simulink model "Control_Model_2020a"  (R2020a)
settings: Solver=ode3  StartTime=0.0  StopTime=20  FixedStep=0.001  RelTol=1e-3
InitFcn:
  | init_parameters
undefined symbols (not defined in the file): Bf, Bm, Br, DiscIntNeverNeededParam, f, g, hg, i_sw, I_tire, Iz, k1, k2, k3, K_LQR, kd_beta, kd_omega, ki_beta, ki_omega, kp_beta, kp_omega, L, Lf, Lm, Lr, m, magnitude, mb, mw, Mz_K, Pn_motor, r, sigbuilder_block, Tn_motor, v_obj, vx0, w0
libraries: simulink x2, Solver_SF x1, simulink_extras x1
(part 2 of 2)

== system Control_Model_2020a/开环驾驶员模型/Sin_(后续可换为轨迹规划结果前向角) ==
  Clock : Clock
  Clock1 : Clock
  Constant : Constant  Value=0
  Constant1 : Constant  Value=0
  Scope : Scope
  Switch : Switch  Criteria=u2 > Threshold  Threshold=3
  Switch1 : Switch  Criteria=u2 > Threshold  Threshold=7
  Transport Delay1 : TransportDelay  DelayTime=3
  rad : Sin  Amplitude=2  Frequency=pi/2  SampleTime=0
  delta_sw : Outport
  wires:
  Constant1/1 -> Switch1/1
  Clock/1 -> Switch/2
  rad/1 -> Transport Delay1/1
  Switch1/1 -> delta_sw/1
  Clock1/1 -> Switch1/2
  Switch/1 -> Switch1/3
  Transport Delay1/1 -> Switch/1, Scope/1
  Constant/1 -> Switch/3

== system Control_Model_2020a/开环驾驶员模型/Step ==
  Step : Step  After=1.4  SampleTime=0
  delta_sw : Outport
  wires:
  Step/1 -> delta_sw/1

== system Control_Model_2020a/7DOF_vehicle/Body/global system transform ==
  vx : Inport
  vy : Inport  Port=2
  wz : Inport  Port=3
  Add : Sum  Inputs=|+-
  Add1 : Sum  Inputs=|++
  Integrator10 : Integrator
  Integrator8 : Integrator
  Integrator9 : Integrator
  Scope : Scope  NumInputPorts=3
  Trigonometric Function1 : Trigonometry
  Trigonometric Function2 : Trigonometry  Operator=cos
  vx*cosr : Product
  vx*sinr : Product
  vy*cosr : Product
  vy*sinr : Product
  x : Outport
  y : Outport  Port=2
  wires:
  vy*cosr/1 -> Add1/2
  Add1/1 -> Scope/2, Integrator9/1
  vx*sinr/1 -> Add1/1
  vx*cosr/1 -> Add/1
  Integrator8/1 -> Scope/1, Trigonometric Function1/1, Trigonometric Function2/1  "r"
  Integrator10/1 -> x/1
  Integrator9/1 -> y/1
  vy/1 -> vy*cosr/1, vy*sinr/1
  wz/1 -> Scope/3, Integrator8/1
  vx/1 -> vx*cosr/1, vx*sinr/1
  vy*sinr/1 -> Add/2
  Trigonometric Function2/1 -> vx*cosr/2, vy*cosr/2
  Add/1 -> Integrator10/1
  Trigonometric Function1/1 -> vx*sinr/2, vy*sinr/2

== system Control_Model_2020a/7DOF_vehicle/Wheel/fl ==
  T_fl : Inport
  Fx_fl : Inport  Port=2
  Fz_fl : Inport  Port=3
  Add : Sum  Inputs=+--
  Constant : Constant  Value=I_tire
  Divide : Product  Inputs=*/
  Gain : Gain  Gain=r
  Gain1 : Gain  Gain=r*f
  Integrator : Integrator  InitialCondition=w0
  w_fl : Outport
  wires:
  Gain/1 -> Add/2
  Fx_fl/1 -> Gain/1
  Fz_fl/1 -> Gain1/1
  T_fl/1 -> Add/1
  Gain1/1 -> Add/3
  Add/1 -> Divide/1
  Constant/1 -> Divide/2
  Divide/1 -> Integrator/1  "dot_w"
  Integrator/1 -> w_fl/1

== system Control_Model_2020a/7DOF_vehicle/Wheel/fr ==
  T_fr : Inport
  Fx_fr : Inport  Port=2
  Fz_fr : Inport  Port=3
  Add : Sum  Inputs=+--
  Constant : Constant  Value=I_tire
  Divide : Product  Inputs=*/
  Gain : Gain  Gain=r
  Gain1 : Gain  Gain=r*f
  Integrator : Integrator  InitialCondition=w0
  w_fr : Outport
  wires:
  Gain1/1 -> Add/3
  Integrator/1 -> w_fr/1
  Divide/1 -> Integrator/1  "dot_w"
  Constant/1 -> Divide/2
  Add/1 -> Divide/1
  Gain/1 -> Add/2
  T_fr/1 -> Add/1
  Fz_fr/1 -> Gain1/1
  Fx_fr/1 -> Gain/1

== system Control_Model_2020a/7DOF_vehicle/Wheel/ml ==
  T_ml : Inport
  Fx_ml : Inport  Port=2
  Fz_ml : Inport  Port=3
  Add : Sum  Inputs=+--
  Constant : Constant  Value=I_tire
  Divide : Product  Inputs=*/
  Gain : Gain  Gain=r
  Gain1 : Gain  Gain=r*f
  Integrator : Integrator  InitialCondition=w0
  w_ml : Outport
  wires:
  Fx_ml/1 -> Gain/1
  Fz_ml/1 -> Gain1/1
  T_ml/1 -> Add/1
  Gain/1 -> Add/2
  Add/1 -> Divide/1
  Constant/1 -> Divide/2
  Divide/1 -> Integrator/1  "dot_w"
  Integrator/1 -> w_ml/1
  Gain1/1 -> Add/3

== system Control_Model_2020a/7DOF_vehicle/Wheel/mr ==
  T_mr : Inport
  Fx_mr : Inport  Port=2
  Fz_mr : Inport  Port=3
  Add : Sum  Inputs=+--
  Constant : Constant  Value=I_tire
  Divide : Product  Inputs=*/
  Gain : Gain  Gain=r
  Gain1 : Gain  Gain=r*f
  Integrator : Integrator  InitialCondition=w0
  w_mr : Outport
  wires:
  Integrator/1 -> w_mr/1
  Divide/1 -> Integrator/1  "dot_w"
  Constant/1 -> Divide/2
  Add/1 -> Divide/1
  Gain/1 -> Add/2
  T_mr/1 -> Add/1
  Fz_mr/1 -> Gain1/1
  Fx_mr/1 -> Gain/1
  Gain1/1 -> Add/3

== system Control_Model_2020a/7DOF_vehicle/Wheel/rl ==
  T_rl : Inport
  Fx_rl : Inport  Port=2
  Fz_rl : Inport  Port=3
  Add : Sum  Inputs=+--
  Constant : Constant  Value=I_tire
  Divide : Product  Inputs=*/
  Gain : Gain  Gain=r
  Gain1 : Gain  Gain=r*f
  Integrator : Integrator  InitialCondition=w0
  w_rl : Outport
  wires:
  Gain1/1 -> Add/3
  Integrator/1 -> w_rl/1
  Divide/1 -> Integrator/1  "dot_w"
  Constant/1 -> Divide/2
  Add/1 -> Divide/1
  Gain/1 -> Add/2
  T_rl/1 -> Add/1
  Fz_rl/1 -> Gain1/1
  Fx_rl/1 -> Gain/1

== system Control_Model_2020a/7DOF_vehicle/Wheel/rr ==
  T_rr : Inport
  Fx_rr : Inport  Port=2
  Fz_rr : Inport  Port=3
  Add : Sum  Inputs=+--
  Constant : Constant  Value=I_tire
  Divide : Product  Inputs=*/
  Gain : Gain  Gain=r
  Gain1 : Gain  Gain=r*f
  Integrator : Integrator  InitialCondition=w0
  w_rr : Outport
  wires:
  Gain1/1 -> Add/3
  Fx_rr/1 -> Gain/1
  Fz_rr/1 -> Gain1/1
  T_rr/1 -> Add/1
  Gain/1 -> Add/2
  Add/1 -> Divide/1
  Constant/1 -> Divide/2
  Divide/1 -> Integrator/1  "dot_w"
  Integrator/1 -> w_rr/1

== system Control_Model_2020a/7DOF_vehicle/alpha_lamda/alpha ==
  vx : Inport
  vy : Inport  Port=2
  wz : Inport  Port=3
  delta_fl : Inport  Port=4
  delta_fr : Inport  Port=5
  Gain{,1..5} (6 alike) : Gain  Gain=-1
  fl : Subsystem
  fr : Subsystem
  ml : Subsystem
  mr : Subsystem
  rl : Subsystem
  rr : Subsystem
  alpha_fl : Outport
  alpha_fr : Outport  Port=2
  alpha_rl : Outport  Port=3
  alpha_rr : Outport  Port=4
  alpha_ml : Outport  Port=5
  alpha_mr : Outport  Port=6
  wires:
  delta_fr/1 -> fr/4(delta_fr)
  delta_fl/1 -> fl/4(delta_fl)
  vy/1 -> rl/2(vy), mr/2(vy), ml/2(vy), fl/2(vy), fr/2(vy), rr/2(vy)
  vx/1 -> rl/1(vx), mr/1(vx), ml/1(vx), fl/1(vx), fr/1(vx), rr/1(vx)
  wz/1 -> rl/3(wz), fr/3(wz), rr/3(wz), mr/3(wz), ml/3(wz), fl/3(wz)
  fl/1(alpha_fl) -> Gain/1
  Gain/1 -> alpha_fl/1
  rl/1(alpha_rl) -> Gain1/1
  Gain1/1 -> alpha_rl/1
  fr/1(alpha_fr) -> Gain2/1
  Gain2/1 -> alpha_fr/1
  rr/1(alpha_rr) -> Gain3/1
  Gain3/1 -> alpha_rr/1
  Gain4/1 -> alpha_ml/1
  Gain5/1 -> alpha_mr/1
  ml/1(alpha_ml) -> Gain4/1
  mr/1(alpha_mr) -> Gain5/1

== system Control_Model_2020a/7DOF_vehicle/alpha_lamda/lamda ==
  vx : Inport
  vy : Inport  Port=2
  wz : Inport  Port=3
  delta_fl : Inport  Port=4
  delta_fr : Inport  Port=5
  w_fl : Inport  Port=6
  w_fr : Inport  Port=7
  w_rl : Inport  Port=8
  w_rr : Inport  Port=9
  w_ml : Inport  Port=10
  w_mr : Inport  Port=11
  fl : Subsystem
  fr : Subsystem
  ml : Subsystem
  mr : Subsystem
  rl : Subsystem
  rr : Subsystem
  lamda_fl : Outport
  lamda_fr : Outport  Port=2
  lamda_rl : Outport  Port=3
  lamda_rr : Outport  Port=4
  lamda_ml : Outport  Port=5
  lamda_mr : Outport  Port=6
  wires:
  fr/1(lamda_fr) -> lamda_fr/1
  rr/1(lamda_rr) -> lamda_rr/1
  w_rl/1 -> rl/1(w_rl)
  w_rr/1 -> rr/1(w_rr)
  w_fr/1 -> fr/1(w_fr)
  delta_fr/1 -> fr/5(delta_fr)
  delta_fl/1 -> fl/5(delta_fl)
  vy/1 -> fl/4(vy), fr/4(vy)
  vx/1 -> fl/3(vx), fr/3(vx), mr/3(vx), rr/3(vx), ml/3(vx), rl/3(vx)
  wz/1 -> fl/2(wz), fr/2(wz), mr/2(wz), rr/2(wz), ml/2(wz), rl/2(wz)
  w_fl/1 -> fl/1(w_fl)
  rl/1(lamda_rl) -> lamda_rl/1
  fl/1(lamda_fl) -> lamda_fl/1
  w_ml/1 -> ml/1(w_ml)
  w_mr/1 -> mr/1(w_mr)
  ml/1(lamda_ml) -> lamda_ml/1
  mr/1(lamda_mr) -> lamda_mr/1

== system Control_Model_2020a/开环驾驶员模型/Sin/Signal Builder ==
  Demux : Demux  Tag=STV Demux  Outputs=1
      settings: DisplayOption=none
  FromWs : FromWorkspace  Tag=STV FromWs  VariableName=tuvar
      SigBuilderData=|
      | common.afterFinalStr = 'Extrapolate'
      | common.sampleTime = 0
      | dataSet.timeRange = [0 10]
      | dataSet.name = 'Group 1'
      | sbobj.Groups.Name = 'Group 1'
      | sbobj.Groups.Signals.Name = 'Signal 1'
      | sbobj.Groups.Signals.XData = [0 1 1.55 2 3 10]
      | sbobj.Groups.Signals.YData = [0 0 294 294 -294 -294]
  Signal 1 : Outport  Tag=STV Outport
  wires:
  Demux/1 -> Signal 1/1
  FromWs/1 -> Demux/1

== system Control_Model_2020a/7DOF_vehicle/alpha_lamda/alpha/fl ==
  vx : Inport
  vy : Inport  Port=2
  wz : Inport  Port=3
  delta_fl : Inport  Port=4
  Add2 : Sum
  Add3 : Sum  Inputs=+-
  Add4 : Sum  Inputs=-+
  Divide : Product  Inputs=/*
  Gain3 : Gain  Gain=Lf
  Gain4 : Gain  Gain=0.5*Bf
  Trigonometric Function : Trigonometry  Operator=atan
  alpha_fl : Outport
  wires:
  wz/1 -> Gain3/1, Gain4/1
  Add4/1 -> alpha_fl/1
  vy/1 -> Add2/1
  delta_fl/1 -> Add4/2
  vx/1 -> Add3/1
  Trigonometric Function/1 -> Add4/1
  Divide/1 -> Trigonometric Function/1
  Add3/1 -> Divide/1
  Add2/1 -> Divide/2
  Gain4/1 -> Add3/2
  Gain3/1 -> Add2/2

== system Control_Model_2020a/7DOF_vehicle/alpha_lamda/alpha/fr ==
  vx : Inport
  vy : Inport  Port=2
  wz : Inport  Port=3
  delta_fr : Inport  Port=4
  Add2 : Sum
  Add3 : Sum
  Add4 : Sum  Inputs=-+
  Divide : Product  Inputs=/*
  Gain3 : Gain  Gain=Lf
  Gain4 : Gain  Gain=0.5*Bf
  Trigonometric Function : Trigonometry  Operator=atan
  alpha_fr : Outport
  wires:
  Gain3/1 -> Add2/2
  Add2/1 -> Divide/2
  Add3/1 -> Divide/1
  Divide/1 -> Trigonometric Function/1
  Trigonometric Function/1 -> Add4/1
  vx/1 -> Add3/1
  delta_fr/1 -> Add4/2
  vy/1 -> Add2/1
  Add4/1 -> alpha_fr/1
  wz/1 -> Gain4/1, Gain3/1
  Gain4/1 -> Add3/2

== system Control_Model_2020a/7DOF_vehicle/alpha_lamda/alpha/ml ==
  vx : Inport
  vy : Inport  Port=2
  wz : Inport  Port=3
  Add2 : Sum  Inputs=+-
  Add3 : Sum  Inputs=+-
  Divide : Product  Inputs=/*
  Gain1 : Gain  Gain=-1
  Gain3 : Gain  Gain=Lm
  Gain4 : Gain  Gain=0.5*Bm
  Trigonometric Function : Trigonometry  Operator=atan
  alpha_ml : Outport
  wires:
  Gain1/1 -> alpha_ml/1
  Gain4/1 -> Add3/2
  Trigonometric Function/1 -> Gain1/1
  wz/1 -> Gain3/1, Gain4/1
  vy/1 -> Add2/1
  vx/1 -> Add3/1
  Divide/1 -> Trigonometric Function/1
  Add3/1 -> Divide/1
  Add2/1 -> Divide/2
  Gain3/1 -> Add2/2

== system Control_Model_2020a/7DOF_vehicle/alpha_lamda/alpha/mr ==
  vx : Inport
  vy : Inport  Port=2
  wz : Inport  Port=3
  Add2 : Sum  Inputs=+-
  Add3 : Sum
  Divide : Product  Inputs=/*
  Gain2 : Gain  Gain=-1
  Gain3 : Gain  Gain=Lm
  Gain4 : Gain  Gain=0.5*Bm
  Trigonometric Function : Trigonometry  Operator=atan
  alpha_mr : Outport
  wires:
  Gain2/1 -> alpha_mr/1
  Gain4/1 -> Add3/2
  Gain3/1 -> Add2/2
  Add2/1 -> Divide/2
  Add3/1 -> Divide/1
  Divide/1 -> Trigonometric Function/1
  vx/1 -> Add3/1
  vy/1 -> Add2/1
  wz/1 -> Gain4/1, Gain3/1
  Trigonometric Function/1 -> Gain2/1

== system Control_Model_2020a/7DOF_vehicle/alpha_lamda/alpha/rl ==
  vx : Inport
  vy : Inport  Port=2
  wz : Inport  Port=3
  Add2 : Sum  Inputs=+-
  Add3 : Sum  Inputs=+-
  Divide : Product  Inputs=/*
  Gain1 : Gain  Gain=-1
  Gain3 : Gain  Gain=Lr
  Gain4 : Gain  Gain=0.5*Br
  Trigonometric Function : Trigonometry  Operator=atan
  alpha_rl : Outport
  wires:
  Gain3/1 -> Add2/2
  Add2/1 -> Divide/2
  Add3/1 -> Divide/1
  Divide/1 -> Trigonometric Function/1
  vx/1 -> Add3/1
  vy/1 -> Add2/1
  wz/1 -> Gain4/1, Gain3/1
  Trigonometric Function/1 -> Gain1/1
  Gain4/1 -> Add3/2
  Gain1/1 -> alpha_rl/1

== system Control_Model_2020a/7DOF_vehicle/alpha_lamda/alpha/rr ==
  vx : Inport
  vy : Inport  Port=2
  wz : Inport  Port=3
  Add2 : Sum  Inputs=+-
  Add3 : Sum
  Divide : Product  Inputs=/*
  Gain2 : Gain  Gain=-1
  Gain3 : Gain  Gain=Lr
  Gain4 : Gain  Gain=0.5*Br
  Trigonometric Function : Trigonometry  Operator=atan
  alpha_rr : Outport
  wires:
  Trigonometric Function/1 -> Gain2/1
  wz/1 -> Gain3/1, Gain4/1
  vy/1 -> Add2/1
  vx/1 -> Add3/1
  Divide/1 -> Trigonometric Function/1
  Add3/1 -> Divide/1
  Add2/1 -> Divide/2
  Gain3/1 -> Add2/2
  Gain4/1 -> Add3/2
  Gain2/1 -> alpha_rr/1

== system Control_Model_2020a/7DOF_vehicle/alpha_lamda/lamda/fl ==
  w_fl : Inport
  wz : Inport  Port=2
  vx : Inport  Port=3
  vy : Inport  Port=4
  delta_fl : Inport  Port=5
  Add1 : Sum  Inputs=-+
  Add2 : Sum
  Add3 : Sum
  Add4 : Sum  Inputs=+-
  Constant1 : Constant  Value=r
  Divide1 : Product  Inputs=**
  Divide2 : Product  Inputs=**
  Divide3 : Product  Inputs=**
  Divide4 : Product  Inputs=/*
  Divide5 : Product  Inputs=*/
  Fcn1 : Fcn  Expr=u+(u==0)*eps
  Gain2 : Gain  Gain=0.5*Bf
  Gain3 : Gain  Gain=Lf
  Saturation : Saturate  UpperLimit=1  LowerLimit=-1
  Switch : Switch  Criteria=u2 > Threshold
  Trigonometric Function1 : Trigonometry
  Trigonometric Function2 : Trigonometry  Operator=cos
  lamda_fl : Outport
  wires:
  Switch/1 -> Saturation/1
  Add3/1 -> Add4/2, Divide5/2  "Vwx_fl"
  Add4/1 -> Switch/2, Divide4/2, Divide5/1
  Divide4/1 -> Switch/1
  Divide5/1 -> Switch/3
  Fcn1/1 -> Divide4/1
  vx/1 -> Add1/2
  Gain2/1 -> Add1/1
  wz/1 -> Gain3/1, Gain2/1
  Add1/1 -> Divide1/1
  delta_fl/1 -> Trigonometric Function2/1, Trigonometric Function1/1
  Trigonometric Function2/1 -> Divide1/2
  vy/1 -> Add2/2
  Gain3/1 -> Add2/1
  Add2/1 -> Divide2/1
  Trigonometric Function1/1 -> Divide2/2
  Divide1/1 -> Add3/1
  Divide2/1 -> Add3/2
  w_fl/1 -> Divide3/1
  Constant1/1 -> Divide3/2
  Divide3/1 -> Add4/1, Fcn1/1  "w*I_tire"
  Saturation/1 -> lamda_fl/1

== system Control_Model_2020a/7DOF_vehicle/alpha_lamda/lamda/fr ==
  w_fr : Inport
  wz : Inport  Port=2
  vx : Inport  Port=3
  vy : Inport  Port=4
  delta_fr : Inport  Port=5
  Add1 : Sum
  Add2 : Sum
  Add3 : Sum
  Add4 : Sum  Inputs=+-
  Constant1 : Constant  Value=r
  Divide1 : Product  Inputs=**
  Divide2 : Product  Inputs=**
  Divide3 : Product  Inputs=**
  Divide4 : Product  Inputs=/*
  Divide5 : Product  Inputs=*/
  Fcn1 : Fcn  Expr=u+(u==0)*eps
  Gain2 : Gain  Gain=0.5*Bf
  Gain3 : Gain  Gain=Lf
  Saturation : Saturate  UpperLimit=1  LowerLimit=-1
  Switch : Switch  Criteria=u2 > Threshold
  Trigonometric Function1 : Trigonometry
  Trigonometric Function2 : Trigonometry  Operator=cos
  lamda_fr : Outport
  wires:
  Saturation/1 -> lamda_fr/1
  vx/1 -> Add1/2
  Gain2/1 -> Add1/1
  wz/1 -> Gain3/1, Gain2/1
  Add1/1 -> Divide1/1
  delta_fr/1 -> Trigonometric Function2/1, Trigonometric Function1/1
  Trigonometric Function2/1 -> Divide1/2
  vy/1 -> Add2/2
  Gain3/1 -> Add2/1
  Add2/1 -> Divide2/1
  Trigonometric Function1/1 -> Divide2/2
  Divide1/1 -> Add3/1
  Divide2/1 -> Add3/2
  w_fr/1 -> Divide3/1
  Constant1/1 -> Divide3/2
  Divide3/1 -> Fcn1/1, Add4/1  "w*I_tire"
  Fcn1/1 -> Divide4/1
  Divide5/1 -> Switch/3
  Divide4/1 -> Switch/1
  Add4/1 -> Divide5/1, Divide4/2, Switch/2
  Add3/1 -> Divide5/2, Add4/2  "Vwx_fr"
  Switch/1 -> Saturation/1

== system Control_Model_2020a/7DOF_vehicle/alpha_lamda/lamda/ml ==
  w_ml : Inport
  wz : Inport  Port=2
  vx : Inport  Port=3
  Add1 : Sum  Inputs=-+
  Add4 : Sum  Inputs=+-
  Constant1 : Constant  Value=r
  Divide3 : Product  Inputs=**
  Divide4 : Product  Inputs=/*
  Divide5 : Product  Inputs=*/
  Fcn1 : Fcn  Expr=u+(u==0)*eps
  Gain2 : Gain  Gain=0.5*Bm
  Saturation : Saturate  UpperLimit=1  LowerLimit=-1
  Switch : Switch  Criteria=u2 > Threshold
  lamda_ml : Outport
  wires:
  Switch/1 -> Saturation/1
  Add1/1 -> Add4/2, Divide5/2
  Add4/1 -> Switch/2, Divide4/2, Divide5/1
  Divide4/1 -> Switch/1
  Divide5/1 -> Switch/3
  Fcn1/1 -> Divide4/1
  Divide3/1 -> Add4/1, Fcn1/1  "w*I_tire"
  Constant1/1 -> Divide3/2
  w_ml/1 -> Divide3/1
  wz/1 -> Gain2/1
  Gain2/1 -> Add1/1
  vx/1 -> Add1/2
  Saturation/1 -> lamda_ml/1

== system Control_Model_2020a/7DOF_vehicle/alpha_lamda/lamda/mr ==
  w_mr : Inport
  wz : Inport  Port=2
  vx : Inport  Port=3
  Add1 : Sum
  Add4 : Sum  Inputs=+-
  Constant1 : Constant  Value=r
  Divide3 : Product  Inputs=**
  Divide4 : Product  Inputs=/*
  Divide5 : Product  Inputs=*/
  Fcn1 : Fcn  Expr=u+(u==0)*eps
  Gain2 : Gain  Gain=0.5*Bm
  Saturation : Saturate  UpperLimit=1  LowerLimit=-1
  Switch : Switch  Criteria=u2 > Threshold
  lamda_mr : Outport
  wires:
  Add1/1 -> Add4/2, Divide5/2  "Vwx_mr"
  Add4/1 -> Switch/2, Divide4/2, Divide5/1
  Divide4/1 -> Switch/1
  Divide5/1 -> Switch/3
  Fcn1/1 -> Divide4/1
  Divide3/1 -> Add4/1, Fcn1/1  "w*I_tire"
  vx/1 -> Add1/2
  Gain2/1 -> Add1/1
  wz/1 -> Gain2/1
  w_mr/1 -> Divide3/1
  Constant1/1 -> Divide3/2
  Switch/1 -> Saturation/1
  Saturation/1 -> lamda_mr/1

== system Control_Model_2020a/7DOF_vehicle/alpha_lamda/lamda/rl ==
  w_rl : Inport
  wz : Inport  Port=2
  vx : Inport  Port=3
  Add1 : Sum  Inputs=-+
  Add4 : Sum  Inputs=+-
  Constant1 : Constant  Value=r
  Divide3 : Product  Inputs=**
  Divide4 : Product  Inputs=/*
  Divide5 : Product  Inputs=*/
  Fcn1 : Fcn  Expr=u+(u==0)*eps
  Gain2 : Gain  Gain=0.5*Br
  Saturation : Saturate  UpperLimit=1  LowerLimit=-1
  Switch : Switch  Criteria=u2 > Threshold
  lamda_rl : Outport
  wires:
  Saturation/1 -> lamda_rl/1
  vx/1 -> Add1/2
  Gain2/1 -> Add1/1
  wz/1 -> Gain2/1
  w_rl/1 -> Divide3/1
  Constant1/1 -> Divide3/2
  Divide3/1 -> Fcn1/1, Add4/1  "w*I_tire"
  Fcn1/1 -> Divide4/1
  Divide5/1 -> Switch/3
  Divide4/1 -> Switch/1
  Add4/1 -> Divide5/1, Divide4/2, Switch/2
  Add1/1 -> Divide5/2, Add4/2
  Switch/1 -> Saturation/1

== system Control_Model_2020a/7DOF_vehicle/alpha_lamda/lamda/rr ==
  w_rr : Inport
  wz : Inport  Port=2
  vx : Inport  Port=3
  Add1 : Sum
  Add4 : Sum  Inputs=+-
  Constant1 : Constant  Value=r
  Divide3 : Product  Inputs=**
  Divide4 : Product  Inputs=/*
  Divide5 : Product  Inputs=*/
  Fcn1 : Fcn  Expr=u+(u==0)*eps
  Gain2 : Gain  Gain=0.5*Br
  Saturation : Saturate  UpperLimit=1  LowerLimit=-1
  Switch : Switch  Criteria=u2 > Threshold
  lamda_rr : Outport
  wires:
  Saturation/1 -> lamda_rr/1
  Switch/1 -> Saturation/1
  Constant1/1 -> Divide3/2
  w_rr/1 -> Divide3/1
  wz/1 -> Gain2/1
  Gain2/1 -> Add1/1
  vx/1 -> Add1/2
  Divide3/1 -> Fcn1/1, Add4/1  "w*I_tire"
  Fcn1/1 -> Divide4/1
  Divide5/1 -> Switch/3
  Divide4/1 -> Switch/1
  Add4/1 -> Divide5/1, Divide4/2, Switch/2
  Add1/1 -> Divide5/2, Add4/2  "Vwx_rr"

== matlab function Control_Model_2020a/Subsystem/Union_Control/MATLAB Function1 ==
  data: u input; B1 output; B2 output
function [B1,B2] = Param_B1B2(u)
if u>=0 && u<0.2
    B1=0.284;B2=2.577;
elseif u>=0.2 && u<0.4
    B1=0.297;B2=3.345;
elseif u>=0.4 && u<0.6
    B1=0.303;B2=4.228;
elseif u>=0.6 && u<0.8
    B1=0.357;B2=4.654;
else 
    B1=0.357;B2=5.573;
end

== matlab function Control_Model_2020a/average_control1/MATLAB Function1 ==
  data: Fz_fl input; Fz_fr input; Fz_rl input; T_fl output; Fz_rr input; T_vx input; M_yaw input; r input; Br input; T_fr output; T_rl output; T_rr output
function [T_fl,T_fr,T_rl,T_rr] = Optimal(Fz_fl,Fz_fr,Fz_rl,Fz_rr,T_vx,M_yaw,r,Br)

T_fl=T_vx/4-M_yaw*r/2/3.2;
T_fr=T_vx/4+M_yaw*r/2/3.2;
T_rl=T_vx/4-M_yaw*r/2/3.2;
T_rr=T_vx/4+M_yaw*r/2/3.2;

== matlab function Control_Model_2020a/Subsystem/Controller_wz/MATLAB Function1 ==
  data: x input; M output
function M=sat(x)
k=5;
d=abs(x/k);
if d<=1
M=x/k;
else
M=sign(x/k);
end

== matlab function Control_Model_2020a/Subsystem/Controller_beta/MATLAB Function1 ==
  data: x input; M output
function M=sat(x)
k=2;
d=abs(x/k);
if d<=1
M=x/k;
else
M=sign(x/k);
end

== matlab function Control_Model_2020a/MPC_Controller/MATLAB Function ==
  data: x input size=[8,1]; delta_u output
function delta_u = fcn(x)
Np =20;     % 预测时域
Nc = 20;     % 控制时域
x_num = 2; % 状态量的个数
u_num = 1; % 控制量的个数
% 参数值，包括：
% 前轴距离质心长度 lf   m
% 后轴距离质心长度 lr   m
% 整车质量 m    kg
% 横摆转动惯量 Iz kg*m^2
lf = 1.02;lr=1.89;m = 1412;Iz=1536.7;
% 前后轴轮胎侧偏刚度 Cf 和 Cr
Cf = -43214*2;Cr = -43214*2;
% 质心侧偏角 x(1)    rad
beta = x(1);
% 横摆角速度 x(2)    rad/s
omega = x(2);
% 前轮转角   x(3)    rad       
delta = x(3);
% 纵向车速 u         m/s
u = x(4);
% 上一周期控制量
u_k_1 = x(8);
% MPC 控制中的状态量与控制量集合
ksi = [beta;omega;u_k_1];

% 二自由度动力学方程得到系统状态转移矩阵 A
a11 = (Cf+Cr)./m/u;
a12 = (Cf*lf-Cr*lr)./m/u^2 - 1;
a21 = (Cf*lf-Cr*lr)./Iz;
a22 = (lf^2*Cf+lr^2*Cr)./Iz/u;

b11 = -Cf/m/u; % *(cos(delta)-delta*sin(delta))
b21 = -lf*Cf/Iz;
A = [a11 a12;a21 a22];
B = [0;1/Iz];
Bcd = [b11;b21];
% 采样时间
T = x(7);
rank = length(A);
% 时间步长 T 进行离散化
G = T*A + eye(rank);
H = T*B;
Bd = T*Bcd;
% 将状态与控制量集合后的增广矩阵
A_ = [G H;zeros(1,2) eye(1)];
B_ = [H;eye(1)];
C_ = [eye(2) zeros(2,1)];
Bd_ = [Bd;0];
% 开始构造 MPC 矩阵（具体原理查看说明文档）
% 构造 MPC 中的 Sc 矩阵（具体原理查看说明文档）
Sc = zeros(Np*x_num,x_num+1);
for i = 1:Np
    Sc((x_num*(i-1)+1):x_num*i,:) = C_*(A_^i);
end
% 构造 MPC 中的 Sd 矩阵（具体原理查看说明文档）
tmp = zeros(x_num,1);
Sd = zeros(Np*x_num,1);
for i = 1:Np
    tmp = tmp + C_*(A_^(i-1))*Bd_;
    Sd((x_num*(i-1)+1):x_num*i) = tmp;
end
% 构造 MPC 中的 Su 矩阵（具体原理查看说明文档）
Su = zeros(Np*x_num,Nc);
for i = 1:Np
    Su_tmp = zeros(x_num,Nc);
    zero_tmp = zeros(x_num,1);
    for j = 1:Nc
        if j<=i
            Su_tmp(:,j) = C_*(A_^(i-j))*B_;
        else
            Su_tmp(:,j) = zero_tmp;
        end
    end
    Su((x_num*(i-1)+1):x_num*i,:) = Su_tmp;
end

% Q 矩阵（权重系数）（具体原理查看说明文档）
Q = zeros(Np*x_num,Np*x_num);
Qi = [0 0;0 10];
zero_tmp = zeros(x_num,x_num);
for i = 1:Np
    Q_tmp = zeros(x_num,Np*x_num);
    for j = 1:Np
        if j==i
            Q_tmp(:,(x_num*(j-1)+1):x_num*j) = Qi;
        else
            Q_tmp(:,(x_num*(j-1)+1):x_num*j) = zero_tmp;
        end
    end
    Q((x_num*(i-1)+1):x_num*i,:) = Q_tmp;
end
% 质心侧偏角与横摆角速度参考值 x(5) 与 x(6)
beta_ref = x(5);
omega_ref = x(6);
Ri = [beta_ref;omega_ref];
Ref = zeros(Np*x_num,1);
% 将当前时刻的参考值设置为整个预测时域内的参考值（可修改为递增模式等）
for i = 1:Np
    %     Ref((2*(i-1)+1):2*i,:) = R_current + (Ri - R_current) * (i/Np);
    Ref((2*(i-1)+1):2*i,:) = Ri; % 期望为恒定值
end
% 计算 MPC 中的关键矩阵
E = Sc*ksi+Sd*delta-Ref;
R = 0.0003*eye(Nc);
H = 2*(Su'*Q'*Q*Su + R'*R);
G = 2*E'*Q'*Q*Su;
% J = 1/2*delta_u'*H*delta_u + G*delta_u;
% 这里用的无约束快速求解方法
% delta_u_arr = zeros(Nm,1);
% [delta_u_arr,~]=quadprog(H,G,[],[]);%计算得到delta_u(m)
%%
delta_u_arr = zeros(Nc,1);
% -inv(H)*G' 直接调用 MPC 简化求解方法，得到控制量
delta_u_arr = -inv(H)*G';
%%
delta_u_tmp = delta_u_arr;
delta_u = delta_u_arr(1);
delta_u = max(-2000,delta_u);
delta_u = min(2000,delta_u);

== matlab function Control_Model_2020a/7DOF_vehicle/pac2002/fl4 ==
  data: Fz input; Fx0 output; camber input; lamda input; alpha input; Fy0 output; Fx output; Fy output; Mz output
function [Fx0,Fy0,Fx,Fy,Mz] = tire(Fz,camber,lamda,alpha)
if Fz>0
%Fz 轮胎垂向载荷 N
%camber 外倾角 rad？？？
%lamda 纵向滑移率
%alpha 车辆侧偏角 rad
alpha=tan(alpha);
camber=sin(camber);
Fz0=4607; %名义垂向载荷N
dfz=(Fz-Fz0)/Fz0;
%% Pure_Fx
%轮胎参数——纵向力
pcx1=1.65;
pdx1=1.3; pdx2=-0.15; pdx3=0;
pex1=0; pex2=0;pex3=0; pex4=0;
pkx1=20; pkx2=0; pkx3=0;
pvx1=0; pvx2=0;
phx1=0; phx2=0;
%pure_Fx 魔术公式
Cx=pcx1;
Shx=phx1+phx2*dfz;
lamda_x=lamda+Shx;
Dx=(pdx1+pdx2*dfz)*(1-pdx3*camber*camber)*Fz;
Ex=(pex1+pex2*dfz+pex3*dfz*dfz)*(1-pex4*sign(lamda_x));
Kx=Fz*(pkx1+pkx2*dfz)*exp(pkx3*dfz);
Bx=Kx/(Cx*Dx);
Svx=Fz*(pvx1+pvx2*dfz);
Fx0=Dx*sin(Cx*atan(Bx*lamda_x-Ex*(Bx*lamda_x-atan(Bx*lamda_x))))+Svx;
%% 联合工况纵向力Fx
%轮胎参数——纵向力
rbx1=20;rbx2=15;
rcx1=1;
rex1=0;rex2=0;
rhx1=0;
%纵向力加权函数
Bxa=rbx1*cos(atan(rbx2*lamda));
Cxa=rcx1;
Exa=rex1+rex2*dfz;
Shxa=rhx1;
alpha_s=alpha+Shxa;
Gxa=cos(Cxa*atan(Bxa*alpha_s-Exa*(Bxa*alpha_s-atan(Bxa*alpha_s))))/cos(Cxa*atan(Bxa*Shxa-Exa*(Bxa*Shxa-atan(Bxa*Shxa))));
Fx=Fx0*Gxa;



%% Pure_Fy
%轮胎参数——侧向力
pcy1=1.529245171;
pdy1=1.038581713; pdy2=-0.179464279; pdy3=-0.683745879;
pey1=-0.39012519; pey2=-0.611160145;pey3=-0.040677215; pey4=-14.95422065;
pky1=-26.056726760; pky2=2.106504624; pky3=0.499984439;
pvy1=0; pvy2=0;pvy3=0;pvy4=0;
phy1=0; phy2=0;phy3=0;
%pure_Fy 魔术公式
Cy=pcy1;
Shy=phy1+phy2*dfz+phy3*camber;
alpha_y=alpha+Shy;
uy=(pdy1+pdy2*dfz)*(1-pdy3*camber*camber);
Dy=uy*Fz;
Ey=(pey1+pey2*dfz)*(1-(pey3+pey4*camber)*sign(alpha_y));
Ky=pky1*Fz0*sin(2*atan(Fz/(pky2*Fz0)))*(1-pky3*abs(camber));
By=Ky/(Cy*Dy);
Svy=Fz*(pvy1+pvy2*dfz+(pvy3+pvy4*dfz)*camber);
Fy0=Dy*sin(Cy*atan(By*alpha_y-Ey*(By*alpha_y-atan(By*alpha_y))))+Svy;
%% 联合工况侧向力Fy
%轮胎参数——侧向力
rby1=10;rby2=10;rby3=-0.027856;
rcy1=1;
rey1=0;rey2=0;
rhy1=0;rhy2=0;
rvy1=0;rvy2=0;rvy3=0;rvy4=20;rvy5=2;rvy6=10;
%侧向力加权函数
Bya=rby1*cos(atan(rby2*(alpha-rby3)));
Cya=rcy1;
Eya=rey1+rey2*dfz;
Shya=rhy1+rhy2*dfz;
lamda_s=lamda+Shya;
Gya=cos(Cya*atan(Bya*lamda_s-Eya*(Bya*lamda_s-atan(Bya*lamda_s))))/cos(Cya*atan(Bya*Shya-Eya*(Bya*Shya-atan(Bya*Shya))));
%轮胎参数——侧向力
Svyr=uy*Fz*(rvy1+rvy2*dfz+rvy3*camber)*cos(atan(rvy4*alpha))*sin(rvy5*atan(rvy6*lamda));
Fy=Fy0*Gya+Svyr;

%% Pure_Mz
%轮胎参数——回正力矩
R0=0.357; %轮胎空载半径/m
qbz1=11.61018865;qbz2=-0.826853524;qbz3=-3.513951124;qbz4=0.063555994;qbz5=-1.014358836;
qcz1=1.064991884;
qdz1=0.091227598;qdz2=-0.001965108;qdz3=0.341001609;qdz4=-3.426482155;
qez1=-9.044014009;qez2=10;qez3=-19.59192084;qez4=0.156693082;qez5=-0.708977656;
%pure_Mz0 魔术公式
Ct=qcz1;
alpha_t=alpha;
Bt=(qbz1+qbz2*dfz+qbz3*dfz^2)*(1+qbz4*camber+qbz5*abs(camber));
Dt=Fz*(qdz1+qdz2*dfz)*(1+qdz3*camber+qdz4*camber^2)*R0/Fz0;
Et=(qez1+qez2*dfz+qez3*dfz^2)*(1+(qez4+qez5*camber)*((2/pi)*atan(Bt*Ct*alpha_t)));
t=Dt*cos(Ct*atan(Bt*alpha_t-Et*(Bt*alpha_t-atan(Bt*alpha_t))))*cos(alpha); %轮胎拖距
%轮胎参数——回正力矩
% qbz9=60;qbz10=1.177895045;
% qdz6=0.000688243;qdz7=0.002750679;qdz8=-0.303576739;qdz9=0.007781541;
%pure_Mz0 魔术公式
% Br=(qbz9+qbz10*By*Cy);
% Cr=1;
% Dr=Fz*(qdz6+qdz7*dfz+(qdz8+qdz9*dfz)*camber)*R0;
% alpha_r=alpha;
%Mzr=Dr*cos(Cr*atan(Br*alpha_r))*cos(alpha); %残余力矩
Mz=-t*Fy0;
else
    Fx0=0;
    Fy0=0;
    Fx=0;
    Fy=0;
    Mz=0;
end

== matlab function Control_Model_2020a/7DOF_vehicle/pac2002/fl5 ==
  data: Fz input; Fx0 output; camber input; lamda input; alpha input; Fy0 output; Fx output; Fy output; Mz output
function [Fx0,Fy0,Fx,Fy,Mz] = tire(Fz,camber,lamda,alpha)
if Fz>0
%Fz 轮胎垂向载荷 N
%camber 外倾角 rad？？？
%lamda 纵向滑移率
%alpha 车辆侧偏角 rad
alpha=tan(alpha);
camber=sin(camber);
Fz0=4607; %名义垂向载荷N
dfz=(Fz-Fz0)/Fz0;
%% Pure_Fx
%轮胎参数——纵向力
pcx1=1.65;
pdx1=1.3; pdx2=-0.15; pdx3=0;
pex1=0; pex2=0;pex3=0; pex4=0;
pkx1=20; pkx2=0; pkx3=0;
pvx1=0; pvx2=0;
phx1=0; phx2=0;
%pure_Fx 魔术公式
Cx=pcx1;
Shx=phx1+phx2*dfz;
lamda_x=lamda+Shx;
Dx=(pdx1+pdx2*dfz)*(1-pdx3*camber*camber)*Fz;
Ex=(pex1+pex2*dfz+pex3*dfz*dfz)*(1-pex4*sign(lamda_x));
Kx=Fz*(pkx1+pkx2*dfz)*exp(pkx3*dfz);
Bx=Kx/(Cx*Dx);
Svx=Fz*(pvx1+pvx2*dfz);
Fx0=Dx*sin(Cx*atan(Bx*lamda_x-Ex*(Bx*lamda_x-atan(Bx*lamda_x))))+Svx;
%% 联合工况纵向力Fx
%轮胎参数——纵向力
rbx1=20;rbx2=15;
rcx1=1;
rex1=0;rex2=0;
rhx1=0;
%纵向力加权函数
Bxa=rbx1*cos(atan(rbx2*lamda));
Cxa=rcx1;
Exa=rex1+rex2*dfz;
Shxa=rhx1;
alpha_s=alpha+Shxa;
Gxa=cos(Cxa*atan(Bxa*alpha_s-Exa*(Bxa*alpha_s-atan(Bxa*alpha_s))))/cos(Cxa*atan(Bxa*Shxa-Exa*(Bxa*Shxa-atan(Bxa*Shxa))));
Fx=Fx0*Gxa;



%% Pure_Fy
%轮胎参数——侧向力
pcy1=1.529245171;
pdy1=1.038581713; pdy2=-0.179464279; pdy3=-0.683745879;
pey1=-0.39012519; pey2=-0.611160145;pey3=-0.040677215; pey4=-14.95422065;
pky1=-26.056726760; pky2=2.106504624; pky3=0.499984439;
pvy1=0; pvy2=0;pvy3=0;pvy4=0;
phy1=0; phy2=0;phy3=0;
%pure_Fy 魔术公式
Cy=pcy1;
Shy=phy1+phy2*dfz+phy3*camber;
alpha_y=alpha+Shy;
uy=(pdy1+pdy2*dfz)*(1-pdy3*camber*camber);
Dy=uy*Fz;
Ey=(pey1+pey2*dfz)*(1-(pey3+pey4*camber)*sign(alpha_y));
Ky=pky1*Fz0*sin(2*atan(Fz/(pky2*Fz0)))*(1-pky3*abs(camber));
By=Ky/(Cy*Dy);
Svy=Fz*(pvy1+pvy2*dfz+(pvy3+pvy4*dfz)*camber);
Fy0=Dy*sin(Cy*atan(By*alpha_y-Ey*(By*alpha_y-atan(By*alpha_y))))+Svy;
%% 联合工况侧向力Fy
%轮胎参数——侧向力
rby1=10;rby2=10;rby3=-0.027856;
rcy1=1;
rey1=0;rey2=0;
rhy1=0;rhy2=0;
rvy1=0;rvy2=0;rvy3=0;rvy4=20;rvy5=2;rvy6=10;
%侧向力加权函数
Bya=rby1*cos(atan(rby2*(alpha-rby3)));
Cya=rcy1;
Eya=rey1+rey2*dfz;
Shya=rhy1+rhy2*dfz;
lamda_s=lamda+Shya;
Gya=cos(Cya*atan(Bya*lamda_s-Eya*(Bya*lamda_s-atan(Bya*lamda_s))))/cos(Cya*atan(Bya*Shya-Eya*(Bya*Shya-atan(Bya*Shya))));
%轮胎参数——侧向力
Svyr=uy*Fz*(rvy1+rvy2*dfz+rvy3*camber)*cos(atan(rvy4*alpha))*sin(rvy5*atan(rvy6*lamda));
Fy=Fy0*Gya+Svyr;

%% Pure_Mz
%轮胎参数——回正力矩
R0=0.357; %轮胎空载半径/m
qbz1=11.61018865;qbz2=-0.826853524;qbz3=-3.513951124;qbz4=0.063555994;qbz5=-1.014358836;
qcz1=1.064991884;
qdz1=0.091227598;qdz2=-0.001965108;qdz3=0.341001609;qdz4=-3.426482155;
qez1=-9.044014009;qez2=10;qez3=-19.59192084;qez4=0.156693082;qez5=-0.708977656;
%pure_Mz0 魔术公式
Ct=qcz1;
alpha_t=alpha;
Bt=(qbz1+qbz2*dfz+qbz3*dfz^2)*(1+qbz4*camber+qbz5*abs(camber));
Dt=Fz*(qdz1+qdz2*dfz)*(1+qdz3*camber+qdz4*camber^2)*R0/Fz0;
Et=(qez1+qez2*dfz+qez3*dfz^2)*(1+(qez4+qez5*camber)*((2/pi)*atan(Bt*Ct*alpha_t)));
t=Dt*cos(Ct*atan(Bt*alpha_t-Et*(Bt*alpha_t-atan(Bt*alpha_t))))*cos(alpha); %轮胎拖距
%轮胎参数——回正力矩
% qbz9=60;qbz10=1.177895045;
% qdz6=0.000688243;qdz7=0.002750679;qdz8=-0.303576739;qdz9=0.007781541;
%pure_Mz0 魔术公式
% Br=(qbz9+qbz10*By*Cy);
% Cr=1;
% Dr=Fz*(qdz6+qdz7*dfz+(qdz8+qdz9*dfz)*camber)*R0;
% alpha_r=alpha;
%Mzr=Dr*cos(Cr*atan(Br*alpha_r))*cos(alpha); %残余力矩
Mz=-t*Fy0;
else
    Fx0=0;
    Fy0=0;
    Fx=0;
    Fy=0;
    Mz=0;
end

== matlab function Control_Model_2020a/7DOF_vehicle/pac2002/fl1 ==
  data: Fz input; Fx0 output; camber input; lamda input; alpha input; Fy0 output; Fx output; Fy output; Mz output
function [Fx0,Fy0,Fx,Fy,Mz] = tire(Fz,camber,lamda,alpha)
if Fz>0
%Fz 轮胎垂向载荷 N
%camber 外倾角 rad？？？
%lamda 纵向滑移率
%alpha 车辆侧偏角 rad
alpha=tan(alpha);
camber=sin(camber);
Fz0=4607; %名义垂向载荷N
dfz=(Fz-Fz0)/Fz0;
%% Pure_Fx
%轮胎参数——纵向力
pcx1=1.65;
pdx1=1.3; pdx2=-0.15; pdx3=0;
pex1=0; pex2=0;pex3=0; pex4=0;
pkx1=20; pkx2=0; pkx3=0;
pvx1=0; pvx2=0;
phx1=0; phx2=0;
%pure_Fx 魔术公式
Cx=pcx1;
Shx=phx1+phx2*dfz;
lamda_x=lamda+Shx;
Dx=(pdx1+pdx2*dfz)*(1-pdx3*camber*camber)*Fz;
Ex=(pex1+pex2*dfz+pex3*dfz*dfz)*(1-pex4*sign(lamda_x));
Kx=Fz*(pkx1+pkx2*dfz)*exp(pkx3*dfz);
Bx=Kx/(Cx*Dx);
Svx=Fz*(pvx1+pvx2*dfz);
Fx0=Dx*sin(Cx*atan(Bx*lamda_x-Ex*(Bx*lamda_x-atan(Bx*lamda_x))))+Svx;
%% 联合工况纵向力Fx
%轮胎参数——纵向力
rbx1=20;rbx2=15;
rcx1=1;
rex1=0;rex2=0;
rhx1=0;
%纵向力加权函数
Bxa=rbx1*cos(atan(rbx2*lamda));
Cxa=rcx1;
Exa=rex1+rex2*dfz;
Shxa=rhx1;
alpha_s=alpha+Shxa;
Gxa=cos(Cxa*atan(Bxa*alpha_s-Exa*(Bxa*alpha_s-atan(Bxa*alpha_s))))/cos(Cxa*atan(Bxa*Shxa-Exa*(Bxa*Shxa-atan(Bxa*Shxa))));
Fx=Fx0*Gxa;



%% Pure_Fy
%轮胎参数——侧向力
pcy1=1.529245171;
pdy1=1.038581713; pdy2=-0.179464279; pdy3=-0.683745879;
pey1=-0.39012519; pey2=-0.611160145;pey3=-0.040677215; pey4=-14.95422065;
pky1=-26.056726760; pky2=2.106504624; pky3=0.499984439;
pvy1=0; pvy2=0;pvy3=0;pvy4=0;
phy1=0; phy2=0;phy3=0;
%pure_Fy 魔术公式
Cy=pcy1;
Shy=phy1+phy2*dfz+phy3*camber;
alpha_y=alpha+Shy;
uy=(pdy1+pdy2*dfz)*(1-pdy3*camber*camber);
Dy=uy*Fz;
Ey=(pey1+pey2*dfz)*(1-(pey3+pey4*camber)*sign(alpha_y));
Ky=pky1*Fz0*sin(2*atan(Fz/(pky2*Fz0)))*(1-pky3*abs(camber));
By=Ky/(Cy*Dy);
Svy=Fz*(pvy1+pvy2*dfz+(pvy3+pvy4*dfz)*camber);
Fy0=Dy*sin(Cy*atan(By*alpha_y-Ey*(By*alpha_y-atan(By*alpha_y))))+Svy;
%% 联合工况侧向力Fy
%轮胎参数——侧向力
rby1=10;rby2=10;rby3=-0.027856;
rcy1=1;
rey1=0;rey2=0;
rhy1=0;rhy2=0;
rvy1=0;rvy2=0;rvy3=0;rvy4=20;rvy5=2;rvy6=10;
%侧向力加权函数
Bya=rby1*cos(atan(rby2*(alpha-rby3)));
Cya=rcy1;
Eya=rey1+rey2*dfz;
Shya=rhy1+rhy2*dfz;
lamda_s=lamda+Shya;
Gya=cos(Cya*atan(Bya*lamda_s-Eya*(Bya*lamda_s-atan(Bya*lamda_s))))/cos(Cya*atan(Bya*Shya-Eya*(Bya*Shya-atan(Bya*Shya))));
%轮胎参数——侧向力
Svyr=uy*Fz*(rvy1+rvy2*dfz+rvy3*camber)*cos(atan(rvy4*alpha))*sin(rvy5*atan(rvy6*lamda));
Fy=Fy0*Gya+Svyr;

%% Pure_Mz
%轮胎参数——回正力矩
R0=0.357; %轮胎空载半径/m
qbz1=11.61018865;qbz2=-0.826853524;qbz3=-3.513951124;qbz4=0.063555994;qbz5=-1.014358836;
qcz1=1.064991884;
qdz1=0.091227598;qdz2=-0.001965108;qdz3=0.341001609;qdz4=-3.426482155;
qez1=-9.044014009;qez2=10;qez3=-19.59192084;qez4=0.156693082;qez5=-0.708977656;
%pure_Mz0 魔术公式
Ct=qcz1;
alpha_t=alpha;
Bt=(qbz1+qbz2*dfz+qbz3*dfz^2)*(1+qbz4*camber+qbz5*abs(camber));
Dt=Fz*(qdz1+qdz2*dfz)*(1+qdz3*camber+qdz4*camber^2)*R0/Fz0;
Et=(qez1+qez2*dfz+qez3*dfz^2)*(1+(qez4+qez5*camber)*((2/pi)*atan(Bt*Ct*alpha_t)));
t=Dt*cos(Ct*atan(Bt*alpha_t-Et*(Bt*alpha_t-atan(Bt*alpha_t))))*cos(alpha); %轮胎拖距
%轮胎参数——回正力矩
% qbz9=60;qbz10=1.177895045;
% qdz6=0.000688243;qdz7=0.002750679;qdz8=-0.303576739;qdz9=0.007781541;
%pure_Mz0 魔术公式
% Br=(qbz9+qbz10*By*Cy);
% Cr=1;
% Dr=Fz*(qdz6+qdz7*dfz+(qdz8+qdz9*dfz)*camber)*R0;
% alpha_r=alpha;
%Mzr=Dr*cos(Cr*atan(Br*alpha_r))*cos(alpha); %残余力矩
Mz=-t*Fy0;
else
    Fx0=0;
    Fy0=0;
    Fx=0;
    Fy=0;
    Mz=0;
end

== matlab function Control_Model_2020a/7DOF_vehicle/pac2002/fl2 ==
  data: Fz input; Fx0 output; camber input; lamda input; alpha input; Fy0 output; Fx output; Fy output; Mz output
function [Fx0,Fy0,Fx,Fy,Mz] = tire(Fz,camber,lamda,alpha)
if Fz>0
%Fz 轮胎垂向载荷 N
%camber 外倾角 rad？？？
%lamda 纵向滑移率
%alpha 车辆侧偏角 rad
alpha=tan(alpha);
camber=sin(camber);
Fz0=4607; %名义垂向载荷N
dfz=(Fz-Fz0)/Fz0;
%% Pure_Fx
%轮胎参数——纵向力
pcx1=1.65;
pdx1=1.3; pdx2=-0.15; pdx3=0;
pex1=0; pex2=0;pex3=0; pex4=0;
pkx1=20; pkx2=0; pkx3=0;
pvx1=0; pvx2=0;
phx1=0; phx2=0;
%pure_Fx 魔术公式
Cx=pcx1;
Shx=phx1+phx2*dfz;
lamda_x=lamda+Shx;
Dx=(pdx1+pdx2*dfz)*(1-pdx3*camber*camber)*Fz;
Ex=(pex1+pex2*dfz+pex3*dfz*dfz)*(1-pex4*sign(lamda_x));
Kx=Fz*(pkx1+pkx2*dfz)*exp(pkx3*dfz);
Bx=Kx/(Cx*Dx);
Svx=Fz*(pvx1+pvx2*dfz);
Fx0=Dx*sin(Cx*atan(Bx*lamda_x-Ex*(Bx*lamda_x-atan(Bx*lamda_x))))+Svx;
%% 联合工况纵向力Fx
%轮胎参数——纵向力
rbx1=20;rbx2=15;
rcx1=1;
rex1=0;rex2=0;
rhx1=0;
%纵向力加权函数
Bxa=rbx1*cos(atan(rbx2*lamda));
Cxa=rcx1;
Exa=rex1+rex2*dfz;
Shxa=rhx1;
alpha_s=alpha+Shxa;
Gxa=cos(Cxa*atan(Bxa*alpha_s-Exa*(Bxa*alpha_s-atan(Bxa*alpha_s))))/cos(Cxa*atan(Bxa*Shxa-Exa*(Bxa*Shxa-atan(Bxa*Shxa))));
Fx=Fx0*Gxa;



%% Pure_Fy
%轮胎参数——侧向力
pcy1=1.529245171;
pdy1=1.038581713; pdy2=-0.179464279; pdy3=-0.683745879;
pey1=-0.39012519; pey2=-0.611160145;pey3=-0.040677215; pey4=-14.95422065;
pky1=-26.056726760; pky2=2.106504624; pky3=0.499984439;
pvy1=0; pvy2=0;pvy3=0;pvy4=0;
phy1=0; phy2=0;phy3=0;
%pure_Fy 魔术公式
Cy=pcy1;
Shy=phy1+phy2*dfz+phy3*camber;
alpha_y=alpha+Shy;
uy=(pdy1+pdy2*dfz)*(1-pdy3*camber*camber);
Dy=uy*Fz;
Ey=(pey1+pey2*dfz)*(1-(pey3+pey4*camber)*sign(alpha_y));
Ky=pky1*Fz0*sin(2*atan(Fz/(pky2*Fz0)))*(1-pky3*abs(camber));
By=Ky/(Cy*Dy);
Svy=Fz*(pvy1+pvy2*dfz+(pvy3+pvy4*dfz)*camber);
Fy0=Dy*sin(Cy*atan(By*alpha_y-Ey*(By*alpha_y-atan(By*alpha_y))))+Svy;
%% 联合工况侧向力Fy
%轮胎参数——侧向力
rby1=10;rby2=10;rby3=-0.027856;
rcy1=1;
rey1=0;rey2=0;
rhy1=0;rhy2=0;
rvy1=0;rvy2=0;rvy3=0;rvy4=20;rvy5=2;rvy6=10;
%侧向力加权函数
Bya=rby1*cos(atan(rby2*(alpha-rby3)));
Cya=rcy1;
Eya=rey1+rey2*dfz;
Shya=rhy1+rhy2*dfz;
lamda_s=lamda+Shya;
Gya=cos(Cya*atan(Bya*lamda_s-Eya*(Bya*lamda_s-atan(Bya*lamda_s))))/cos(Cya*atan(Bya*Shya-Eya*(Bya*Shya-atan(Bya*Shya))));
%轮胎参数——侧向力
Svyr=uy*Fz*(rvy1+rvy2*dfz+rvy3*camber)*cos(atan(rvy4*alpha))*sin(rvy5*atan(rvy6*lamda));
Fy=Fy0*Gya+Svyr;

%% Pure_Mz
%轮胎参数——回正力矩
R0=0.357; %轮胎空载半径/m
qbz1=11.61018865;qbz2=-0.826853524;qbz3=-3.513951124;qbz4=0.063555994;qbz5=-1.014358836;
qcz1=1.064991884;
qdz1=0.091227598;qdz2=-0.001965108;qdz3=0.341001609;qdz4=-3.426482155;
qez1=-9.044014009;qez2=10;qez3=-19.59192084;qez4=0.156693082;qez5=-0.708977656;
%pure_Mz0 魔术公式
Ct=qcz1;
alpha_t=alpha;
Bt=(qbz1+qbz2*dfz+qbz3*dfz^2)*(1+qbz4*camber+qbz5*abs(camber));
Dt=Fz*(qdz1+qdz2*dfz)*(1+qdz3*camber+qdz4*camber^2)*R0/Fz0;
Et=(qez1+qez2*dfz+qez3*dfz^2)*(1+(qez4+qez5*camber)*((2/pi)*atan(Bt*Ct*alpha_t)));
t=Dt*cos(Ct*atan(Bt*alpha_t-Et*(Bt*alpha_t-atan(Bt*alpha_t))))*cos(alpha); %轮胎拖距
%轮胎参数——回正力矩
% qbz9=60;qbz10=1.177895045;
% qdz6=0.000688243;qdz7=0.002750679;qdz8=-0.303576739;qdz9=0.007781541;
%pure_Mz0 魔术公式
% Br=(qbz9+qbz10*By*Cy);
% Cr=1;
% Dr=Fz*(qdz6+qdz7*dfz+(qdz8+qdz9*dfz)*camber)*R0;
% alpha_r=alpha;
%Mzr=Dr*cos(Cr*atan(Br*alpha_r))*cos(alpha); %残余力矩
Mz=-t*Fy0;
else
    Fx0=0;
    Fy0=0;
    Fx=0;
    Fy=0;
    Mz=0;
end

== matlab function Control_Model_2020a/7DOF_vehicle/pac2002/fl ==
  data: Fz input; Fx0 output; camber input; lamda input; alpha input; Fy0 output; Fx output; Fy output; Mz output
function [Fx0,Fy0,Fx,Fy,Mz] = tire(Fz,camber,lamda,alpha)
if Fz>0
%Fz 轮胎垂向载荷 N
%camber 外倾角 rad？？？
%lamda 纵向滑移率
%alpha 车辆侧偏角 rad
alpha=tan(alpha);
camber=sin(camber);
Fz0=4607; %名义垂向载荷N
dfz=(Fz-Fz0)/Fz0;
%% Pure_Fx
%轮胎参数——纵向力
pcx1=1.65;
pdx1=1.3; pdx2=-0.15; pdx3=0;
pex1=0; pex2=0;pex3=0; pex4=0;
pkx1=20; pkx2=0; pkx3=0;
pvx1=0; pvx2=0;
phx1=0; phx2=0;
%pure_Fx 魔术公式
Cx=pcx1;
Shx=phx1+phx2*dfz;
lamda_x=lamda+Shx;
Dx=(pdx1+pdx2*dfz)*(1-pdx3*camber*camber)*Fz;
Ex=(pex1+pex2*dfz+pex3*dfz*dfz)*(1-pex4*sign(lamda_x));
Kx=Fz*(pkx1+pkx2*dfz)*exp(pkx3*dfz);
Bx=Kx/(Cx*Dx);
Svx=Fz*(pvx1+pvx2*dfz);
Fx0=Dx*sin(Cx*atan(Bx*lamda_x-Ex*(Bx*lamda_x-atan(Bx*lamda_x))))+Svx;
%% 联合工况纵向力Fx
%轮胎参数——纵向力
rbx1=20;rbx2=15;
rcx1=1;
rex1=0;rex2=0;
rhx1=0;
%纵向力加权函数
Bxa=rbx1*cos(atan(rbx2*lamda));
Cxa=rcx1;
Exa=rex1+rex2*dfz;
Shxa=rhx1;
alpha_s=alpha+Shxa;
Gxa=cos(Cxa*atan(Bxa*alpha_s-Exa*(Bxa*alpha_s-atan(Bxa*alpha_s))))/cos(Cxa*atan(Bxa*Shxa-Exa*(Bxa*Shxa-atan(Bxa*Shxa))));
Fx=Fx0*Gxa;



%% Pure_Fy
%轮胎参数——侧向力
pcy1=1.529245171;
pdy1=1.038581713; pdy2=-0.179464279; pdy3=-0.683745879;
pey1=-0.39012519; pey2=-0.611160145;pey3=-0.040677215; pey4=-14.95422065;
pky1=-26.056726760; pky2=2.106504624; pky3=0.499984439;
pvy1=0; pvy2=0;pvy3=0;pvy4=0;
phy1=0; phy2=0;phy3=0;
%pure_Fy 魔术公式
Cy=pcy1;
Shy=phy1+phy2*dfz+phy3*camber;
alpha_y=alpha+Shy;
uy=(pdy1+pdy2*dfz)*(1-pdy3*camber*camber);
Dy=uy*Fz;
Ey=(pey1+pey2*dfz)*(1-(pey3+pey4*camber)*sign(alpha_y));
Ky=pky1*Fz0*sin(2*atan(Fz/(pky2*Fz0)))*(1-pky3*abs(camber));
By=Ky/(Cy*Dy);
Svy=Fz*(pvy1+pvy2*dfz+(pvy3+pvy4*dfz)*camber);
Fy0=Dy*sin(Cy*atan(By*alpha_y-Ey*(By*alpha_y-atan(By*alpha_y))))+Svy;
%% 联合工况侧向力Fy
%轮胎参数——侧向力
rby1=10;rby2=10;rby3=-0.027856;
rcy1=1;
rey1=0;rey2=0;
rhy1=0;rhy2=0;
rvy1=0;rvy2=0;rvy3=0;rvy4=20;rvy5=2;rvy6=10;
%侧向力加权函数
Bya=rby1*cos(atan(rby2*(alpha-rby3)));
Cya=rcy1;
Eya=rey1+rey2*dfz;
Shya=rhy1+rhy2*dfz;
lamda_s=lamda+Shya;
Gya=cos(Cya*atan(Bya*lamda_s-Eya*(Bya*lamda_s-atan(Bya*lamda_s))))/cos(Cya*atan(Bya*Shya-Eya*(Bya*Shya-atan(Bya*Shya))));
%轮胎参数——侧向力
Svyr=uy*Fz*(rvy1+rvy2*dfz+rvy3*camber)*cos(atan(rvy4*alpha))*sin(rvy5*atan(rvy6*lamda));
Fy=Fy0*Gya+Svyr;

%% Pure_Mz
%轮胎参数——回正力矩
R0=0.357; %轮胎空载半径/m
qbz1=11.61018865;qbz2=-0.826853524;qbz3=-3.513951124;qbz4=0.063555994;qbz5=-1.014358836;
qcz1=1.064991884;
qdz1=0.091227598;qdz2=-0.001965108;qdz3=0.341001609;qdz4=-3.426482155;
qez1=-9.044014009;qez2=10;qez3=-19.59192084;qez4=0.156693082;qez5=-0.708977656;
%pure_Mz0 魔术公式
Ct=qcz1;
alpha_t=alpha;
Bt=(qbz1+qbz2*dfz+qbz3*dfz^2)*(1+qbz4*camber+qbz5*abs(camber));
Dt=Fz*(qdz1+qdz2*dfz)*(1+qdz3*camber+qdz4*camber^2)*R0/Fz0;
Et=(qez1+qez2*dfz+qez3*dfz^2)*(1+(qez4+qez5*camber)*((2/pi)*atan(Bt*Ct*alpha_t)));
t=Dt*cos(Ct*atan(Bt*alpha_t-Et*(Bt*alpha_t-atan(Bt*alpha_t))))*cos(alpha); %轮胎拖距
%轮胎参数——回正力矩
% qbz9=60;qbz10=1.177895045;
% qdz6=0.000688243;qdz7=0.002750679;qdz8=-0.303576739;qdz9=0.007781541;
%pure_Mz0 魔术公式
% Br=(qbz9+qbz10*By*Cy);
% Cr=1;
% Dr=Fz*(qdz6+qdz7*dfz+(qdz8+qdz9*dfz)*camber)*R0;
% alpha_r=alpha;
%Mzr=Dr*cos(Cr*atan(Br*alpha_r))*cos(alpha); %残余力矩
Mz=-t*Fy0;
else
    Fx0=0;
    Fy0=0;
    Fx=0;
    Fy=0;
    Mz=0;
end

== matlab function Control_Model_2020a/7DOF_vehicle/pac2002/fl3 ==
  data: Fz input; Fx0 output; camber input; lamda input; alpha input; Fy0 output; Fx output; Fy output; Mz output
function [Fx0,Fy0,Fx,Fy,Mz] = tire(Fz,camber,lamda,alpha)
if Fz>0
%Fz 轮胎垂向载荷 N
%camber 外倾角 rad？？？
%lamda 纵向滑移率
%alpha 车辆侧偏角 rad
alpha=tan(alpha);
camber=sin(camber);
Fz0=4607; %名义垂向载荷N
dfz=(Fz-Fz0)/Fz0;
%% Pure_Fx
%轮胎参数——纵向力
pcx1=1.65;
pdx1=1.3; pdx2=-0.15; pdx3=0;
pex1=0; pex2=0;pex3=0; pex4=0;
pkx1=20; pkx2=0; pkx3=0;
pvx1=0; pvx2=0;
phx1=0; phx2=0;
%pure_Fx 魔术公式
Cx=pcx1;
Shx=phx1+phx2*dfz;
lamda_x=lamda+Shx;
Dx=(pdx1+pdx2*dfz)*(1-pdx3*camber*camber)*Fz;
Ex=(pex1+pex2*dfz+pex3*dfz*dfz)*(1-pex4*sign(lamda_x));
Kx=Fz*(pkx1+pkx2*dfz)*exp(pkx3*dfz);
Bx=Kx/(Cx*Dx);
Svx=Fz*(pvx1+pvx2*dfz);
Fx0=Dx*sin(Cx*atan(Bx*lamda_x-Ex*(Bx*lamda_x-atan(Bx*lamda_x))))+Svx;
%% 联合工况纵向力Fx
%轮胎参数——纵向力
rbx1=20;rbx2=15;
rcx1=1;
rex1=0;rex2=0;
rhx1=0;
%纵向力加权函数
Bxa=rbx1*cos(atan(rbx2*lamda));
Cxa=rcx1;
Exa=rex1+rex2*dfz;
Shxa=rhx1;
alpha_s=alpha+Shxa;
Gxa=cos(Cxa*atan(Bxa*alpha_s-Exa*(Bxa*alpha_s-atan(Bxa*alpha_s))))/cos(Cxa*atan(Bxa*Shxa-Exa*(Bxa*Shxa-atan(Bxa*Shxa))));
Fx=Fx0*Gxa;



%% Pure_Fy
%轮胎参数——侧向力
pcy1=1.529245171;
pdy1=1.038581713; pdy2=-0.179464279; pdy3=-0.683745879;
pey1=-0.39012519; pey2=-0.611160145;pey3=-0.040677215; pey4=-14.95422065;
pky1=-26.056726760; pky2=2.106504624; pky3=0.499984439;
pvy1=0; pvy2=0;pvy3=0;pvy4=0;
phy1=0; phy2=0;phy3=0;
%pure_Fy 魔术公式
Cy=pcy1;
Shy=phy1+phy2*dfz+phy3*camber;
alpha_y=alpha+Shy;
uy=(pdy1+pdy2*dfz)*(1-pdy3*camber*camber);
Dy=uy*Fz;
Ey=(pey1+pey2*dfz)*(1-(pey3+pey4*camber)*sign(alpha_y));
Ky=pky1*Fz0*sin(2*atan(Fz/(pky2*Fz0)))*(1-pky3*abs(camber));
By=Ky/(Cy*Dy);
Svy=Fz*(pvy1+pvy2*dfz+(pvy3+pvy4*dfz)*camber);
Fy0=Dy*sin(Cy*atan(By*alpha_y-Ey*(By*alpha_y-atan(By*alpha_y))))+Svy;
%% 联合工况侧向力Fy
%轮胎参数——侧向力
rby1=10;rby2=10;rby3=-0.027856;
rcy1=1;
rey1=0;rey2=0;
rhy1=0;rhy2=0;
rvy1=0;rvy2=0;rvy3=0;rvy4=20;rvy5=2;rvy6=10;
%侧向力加权函数
Bya=rby1*cos(atan(rby2*(alpha-rby3)));
Cya=rcy1;
Eya=rey1+rey2*dfz;
Shya=rhy1+rhy2*dfz;
lamda_s=lamda+Shya;
Gya=cos(Cya*atan(Bya*lamda_s-Eya*(Bya*lamda_s-atan(Bya*lamda_s))))/cos(Cya*atan(Bya*Shya-Eya*(Bya*Shya-atan(Bya*Shya))));
%轮胎参数——侧向力
Svyr=uy*Fz*(rvy1+rvy2*dfz+rvy3*camber)*cos(atan(rvy4*alpha))*sin(rvy5*atan(rvy6*lamda));
Fy=Fy0*Gya+Svyr;

%% Pure_Mz
%轮胎参数——回正力矩
R0=0.357; %轮胎空载半径/m
qbz1=11.61018865;qbz2=-0.826853524;qbz3=-3.513951124;qbz4=0.063555994;qbz5=-1.014358836;
qcz1=1.064991884;
qdz1=0.091227598;qdz2=-0.001965108;qdz3=0.341001609;qdz4=-3.426482155;
qez1=-9.044014009;qez2=10;qez3=-19.59192084;qez4=0.156693082;qez5=-0.708977656;
%pure_Mz0 魔术公式
Ct=qcz1;
alpha_t=alpha;
Bt=(qbz1+qbz2*dfz+qbz3*dfz^2)*(1+qbz4*camber+qbz5*abs(camber));
Dt=Fz*(qdz1+qdz2*dfz)*(1+qdz3*camber+qdz4*camber^2)*R0/Fz0;
Et=(qez1+qez2*dfz+qez3*dfz^2)*(1+(qez4+qez5*camber)*((2/pi)*atan(Bt*Ct*alpha_t)));
t=Dt*cos(Ct*atan(Bt*alpha_t-Et*(Bt*alpha_t-atan(Bt*alpha_t))))*cos(alpha); %轮胎拖距
%轮胎参数——回正力矩
% qbz9=60;qbz10=1.177895045;
% qdz6=0.000688243;qdz7=0.002750679;qdz8=-0.303576739;qdz9=0.007781541;
%pure_Mz0 魔术公式
% Br=(qbz9+qbz10*By*Cy);
% Cr=1;
% Dr=Fz*(qdz6+qdz7*dfz+(qdz8+qdz9*dfz)*camber)*R0;
% alpha_r=alpha;
%Mzr=Dr*cos(Cr*atan(Br*alpha_r))*cos(alpha); %残余力矩
Mz=-t*Fy0;
else
    Fx0=0;
    Fy0=0;
    Fx=0;
    Fy=0;
    Mz=0;
end

== matlab function Control_Model_2020a/MATLAB Function ==
  data: vx input; delta input; u input; wz_exp output; beta_exp output
function [wz_exp,beta_exp] = Two_dof(vx,delta,u)
% m = 6545; %整车质量kg,oral:1412
% mb = 4455; %车身质量kg,oral:1400
% mw = (m-mb)/6; %轮胎重力kg,6 kg/p
% Bf = 2.03; %前轴轮距m
% Bm = 1.863; 
% Br = 1.863; %后轴轮距m 1.55
% Lf = 1.25; %质心距离前轴的距离m 
% Lm = 1.98;
% Lr = 5.25; %质心距离后轴的距离m
% L = Lf+Lm+Lr; %轴距m
m = 6545; %整车质量kg,oral:1412
Lf = 1.25; %质心距离前轴的距离m 
Lm = 1.98;
Lr = 5.25; %质心距离后轴的距离m
L = Lf+Lm+Lr;
% k1=-160e3;%两前轮侧偏刚度之和 N/rad  kf
% k2=-160e3;%两后轮侧偏刚度之和 N/ra  km
% k3=-160e3;%两中轮侧偏刚度之和 N/rad   kr

k1 = -111378;%%两前轮侧偏刚度之和 N/rad
k2 = -175160;%%两后轮侧偏刚度之和 N/rad
k3 = -321663;%%两后轮侧偏刚度之和 N/rad

% c1=k1*L/(m*Lr); %侧偏系数 1/rad
% c2=k2*L/(m*Lf);
% K=-(1/c1-1/c2)/L;
% wz_exp = (min(abs(vx*delta/(L*(1+K*vx^2))),abs(0.85*u*9.8/vx)))*sign(delta);
% beta_exp= (min(abs(((Lr/L+m*Lf*vx^2/(L^2*k1))/(1+K*vx^2))*delta),abs(u*9.8*(Lr/vx^2+m*Lf/k2/L))))*sign(((Lr/L+m*Lf*vx^2/(L^2*k1))/(1+K*vx^2))*delta);
K=k1*k3*(Lf+Lr)^2+k3*(k1*(Lf^2-Lm^2)+k3*(Lr^2-Lm^2))+m*vx^2*(Lf*k1-Lm*k2-Lr*k3);
wz_exp = (min(abs(k1*((Lf+Lm)*k2+(Lf+Lr)*k3)*vx*delta/K),abs(0.85*u*9.8/vx)))*sign(delta);
beta_exp = (min(abs(((Lf+Lr)*(Lm+Lr)*k1*delta+k1*delta*Lf*m*vx^2-Lm*k1*((Lf+Lm)*k2+(Lf+Lr)*k3)*delta)/K),abs(((Lf+Lr)*(Lm+Lr)*k1*delta+k1*delta*Lf*m*vx^2)/K-0.85*u*9.8*Lm/vx^2)))*sign(((Lf+Lr)*(Lm+Lr)*k1*delta+k1*delta*Lf*m*vx^2-Lm*k1*((Lf+Lm)*k2+(Lf+Lr)*k3)*delta)/K);

== matlab function Control_Model_2020a/optimal_control/MATLAB Function1 ==
  data: Fz_fl input; Fz_fr input; Fz_rl input; T_fl output; Fz_rr input; Fz_ml input; Fz_mr input; T_vx input; M_yaw input; r input; Br input; T_fr output; T_rl output; T_rr output; T_ml output; T_mr output
function [T_fl,T_fr,T_rl,T_rr,T_ml,T_mr] = Optimal(Fz_fl,Fz_fr,Fz_rl,Fz_rr,Fz_ml,Fz_mr,T_vx,M_yaw,r,Br)
%u为路面附着系数
% a1=2*u^2*(Fz_fl^2+Fz_rl^2);
% a2=2*u^2*(Fz_fr^2+Fz_rr^2);
% b1=Fz_rl^2*T_vx/2*r^2-Fz_rl^2*M_yaw/Br*r^3;
% b2=Fz_rr^2*T_vx/2*r^2+Fz_rr^2*M_yaw/Br*r^3;
% T_rl=b1/a1;
% T_rr=b2/a2;
% T_fl=T_vx/2-M_yaw/Br*r-T_rl;
% T_fr=T_vx/2+M_yaw/Br*r-T_rr;

a1=Fz_fl^2*Fz_rl^2+Fz_fl^2*Fz_ml^2+4*Fz_rl^2*Fz_ml^2;
a2=Fz_fr^2*Fz_rr^2+Fz_fr^2*Fz_mr^2+4*Fz_rr^2*Fz_mr^2;
b1=Fz_rl^2*Fz_ml^2*(T_vx-2*M_yaw/Br*r);
b2=Fz_rr^2*Fz_mr^2*(T_vx+2*M_yaw/Br*r);
T_rl=b1/a1;
T_rr=b2/a2;
T_fl=T_vx/2-M_yaw/Br*r-2*T_rl;
T_fr=T_vx/2+M_yaw/Br*r-2*T_rr;
T_ml=T_rl;
T_mr=T_rr;
